simulink model "aerosonde_dist"  (Simulink 5.0)
settings: Solver=ode4  SolverMode=SingleTasking  StartTime=0.0  StopTime=200  FixedStep=0.008  RelTol=1e-3
libraries: simulink_extras x3, aerosimlib x2
settings Model: LastModifiedBy=jonathan How  SaveTime=off  SaveOutput=off  LimitDataPoints=off  UnconnectedInputMsg=none  UnconnectedOutputMsg=none  UnconnectedLineMsg=none  BlockReductionOpt=off  BooleanDataType=off

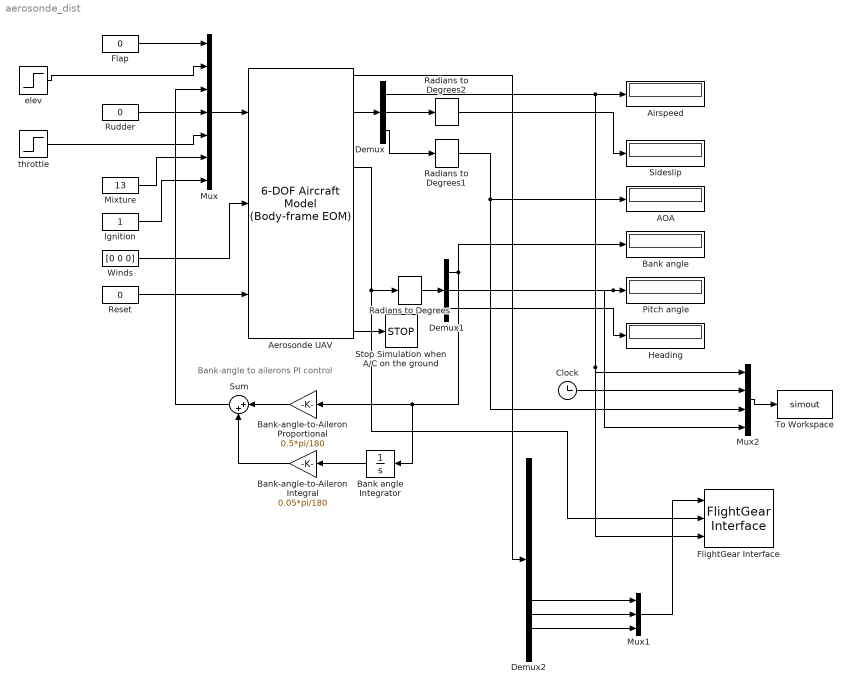
== system aerosonde_dist ==
  note: Bank-angle to ailerons PI control
  AOA : Display
  Aerosonde UAV : aerosimlib/Complete Aircraft/6-DOF Aircraft Model (Body-frame EOM)  aircraftcfg='aerosondecfg.mat'  VelocitiesIni=[23 0 0]'  RatesIni=[0 0 0]'  QuaternionsIni=[1 0 0 0]'  PositionIni=[45*pi/180 -122*pi/180 1000]'  FuelIni=2  OmegaIni=5000*pi/30  GndAlt=20  wmmfile='C:\Program Files\AeroSim\wmm.cof'  dmy=[11 25 2004]  tsamp=0.008
  Airspeed : Display
  Bank angle : Display
  Bank angle Integrator : Integrator  Orientation=left
  Bank-angle-to-Aileron Integral : Gain  Orientation=left  Gain=0.05*pi/180  SaturateOnIntegerOverflow=on
  Bank-angle-to-Aileron Proportional : Gain  Orientation=left  Gain=0.5*pi/180  SaturateOnIntegerOverflow=on
  Clock : Clock
      settings: Decimation=10
  Demux : Demux  Outputs=3
  Demux1 : Demux  Outputs=3
  Demux2 : Demux  Outputs=15
  Flap : Constant  Value=0
  FlightGear Interface : aerosimlib/Pilot Interface/FlightGear Interface  hostname='localhost'  tsamp=0.016
  Heading : Display
  Ignition : Constant
  Mixture : Constant  Value=13
  Mux : Mux  Inputs=7
  Mux1 : Mux  Inputs=3
  Mux2 : Mux
  Pitch angle : Display
  Radians to Degrees : simulink_extras/Transformations/Radians to Degrees
  Radians to Degrees1 : simulink_extras/Transformations/Radians to Degrees
  Radians to Degrees2 : simulink_extras/Transformations/Radians to Degrees
  Reset : Constant  Value=0
  Rudder : Constant  Value=0
  Sideslip : Display
  Stop Simulation when A/C on the ground : Stop
  Sum : Sum  Orientation=left  Inputs=|++  SaturateOnIntegerOverflow=on  InputSameDT=on
  To Workspace : ToWorkspace  VariableName=simout  SampleTime=-1  SaveFormat=Array
  Winds : Constant  Value=[0 0 0]
  elev : Step  Time=100  After=0*pi/180  SampleTime=0
  throttle : Step  Time=100  Before=.5  After=.8  SampleTime=0
  wires:
  Reset/1 -> Aerosonde UAV/3
  Winds/1 -> Aerosonde UAV/2
  Aerosonde UAV/1 -> Demux2/1
  Aerosonde UAV/6 -> FlightGear Interface/2, Radians to Degrees/1
  Aerosonde UAV/3 -> Demux/1
  Demux/3 -> Radians to Degrees1/1
  Demux/2 -> Radians to Degrees2/1
  Demux/1 -> Airspeed/1, Mux2/1, FlightGear Interface/3
  Radians to Degrees2/1 -> Sideslip/1
  Aerosonde UAV/15 -> Stop Simulation when A/C on the ground/1
  Radians to Degrees/1 -> Demux1/1
  Demux1/2 -> Pitch angle/1, Mux2/4
  Demux1/3 -> Heading/1
  Demux1/1 -> Bank angle/1, Bank-angle-to-Aileron Proportional/1, Bank angle Integrator/1
  Flap/1 -> Mux/1
  Rudder/1 -> Mux/4
  Mixture/1 -> Mux/6
  Ignition/1 -> Mux/7
  Mux/1 -> Aerosonde UAV/1
  Bank-angle-to-Aileron Proportional/1 -> Sum/1
  Bank angle Integrator/1 -> Bank-angle-to-Aileron Integral/1
  Bank-angle-to-Aileron Integral/1 -> Sum/2
  Mux1/1 -> FlightGear Interface/1
  Demux2/11 -> Mux1/1
  Demux2/12 -> Mux1/2
  Demux2/13 -> Mux1/3
  Sum/1 -> Mux/3
  Clock/1 -> Mux2/2
  Mux2/1 -> To Workspace/1
  Radians to Degrees1/1 -> Mux2/3, AOA/1
  throttle/1 -> Mux/5
  elev/1 -> Mux/2
